simulink model "HW2_adarbha_sim"  (Simulink 7.7)
settings: Solver=ode45  StartTime=0.0  StopTime=time_end  RelTol=1e-3
PreLoadFcn:
  | HW2_adarbha
InitFcn:
  | HW2_adarbha
undefined symbols (not defined in the file): Area, Cd, density, mass, slope_deg, time_s, time_s_slope, vel_mph, weight_N
libraries: simulink x1
settings Model: Creator=Arjun  LastModifiedBy=Arjun

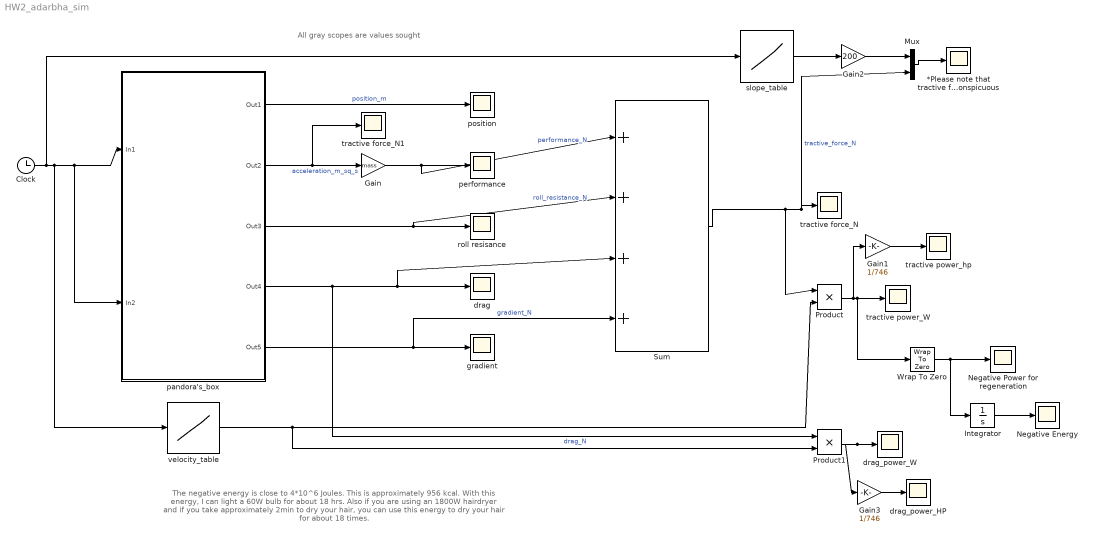
== system HW2_adarbha_sim ==
  note: The negative energy is close to 4*10^6 Joules. This is approximately 956 kcal. With this energy, I can light a 60W bulb for about 18 hrs.
      | Also if you are using an 1800W hairdryer and if you take approximately 2min to dry your hair, you can use this energy to dry your hair for about 18 times.
  note: All gray scopes are values sought
  *Please note that tractive force and slope are on the same axis but slope is multiplied by a factor of 200 so that the variation is conspicuous : Scope
      settings: SaveName=ScopeData13
  Clock : Clock
      settings: Decimation=10
  Gain : Gain  Gain=mass
  Gain1 : Gain  Gain=1/746
  Gain2 : Gain  Gain=200
  Gain3 : Gain  Gain=1/746
  Integrator : Integrator
  Mux : Mux  Inputs=2
  Negative Energy : Scope
      settings: SaveName=power_regen1  DataFormat=Array
  Negative Power for regeneration : Scope
      settings: SaveName=power_regen  DataFormat=Array
  Product : Product  RndMeth=Zero
  Product1 : Product  RndMeth=Zero
  Sum : Sum  Inputs=|++++
  Wrap To Zero : simulink/Discontinuities/Wrap To Zero  SystemSampleTime=-1  Threshold=0
  drag : Scope
      settings: SaveName=ScopeData4
  drag_power_HP : Scope
      settings: SaveName=ScopeData10
  drag_power_W : Scope
      settings: SaveName=ScopeData9
  gradient : Scope
      settings: SaveName=ScopeData5
  pandora's_box : Subsystem
  performance : Scope
      settings: SaveName=ScopeData6
  position : Scope
      settings: SaveName=ScopeData2
  roll resisance : Scope
      settings: SaveName=ScopeData3
  slope_table : Lookup_n-D  NumberOfTableDimensions=1  BreakpointsForDimension1=time_s_slope  Table=slope_deg  RndMeth=Simplest  InputSameDT=on
  tractive force_N : Scope
      settings: SaveName=ScopeData7
  tractive force_N1 : Scope
      settings: SaveName=ScopeData11
  tractive power_W : Scope
      settings: SaveName=ScopeData8
  tractive power_hp : Scope
      settings: SaveName=tractive_power  DataFormat=Array
  velocity_table : Lookup_n-D  NumberOfTableDimensions=1  BreakpointsForDimension1=time_s  Table=vel_mph  RndMeth=Simplest  InputSameDT=on
  wires:
  Clock/1 -> pandora's_box/2(In2), pandora's_box/1(In1), velocity_table/1, slope_table/1
  pandora's_box/2(Out2) -> Gain/1, tractive force_N1/1  "acceleration_m_sq_s"
  pandora's_box/1(Out1) -> position/1  "position_m"
  pandora's_box/4(Out4) -> drag/1, Sum/3, Product1/1  "drag_N"
  pandora's_box/5(Out5) -> gradient/1, Sum/4  "gradient_N"
  pandora's_box/3(Out3) -> roll resisance/1, Sum/2  "roll_resistance_N"
  Gain/1 -> performance/1, Sum/1  "performance_N"
  Sum/1 -> Product/1, tractive force_N/1, Mux/2  "tractive_force_N"
  velocity_table/1 -> Product/2, Product1/2
  Product/1 -> Gain1/1, tractive power_W/1, Wrap To Zero/1
  Product1/1 -> drag_power_W/1, Gain3/1
  Gain1/1 -> tractive power_hp/1
  Wrap To Zero/1 -> Negative Power for regeneration/1, Integrator/1
  Mux/1 -> *Please note that tractive force and slope are on the same axis but slope is multiplied by a factor of 200 so that the variation is conspicuous/1
  slope_table/1 -> Gain2/1
  Gain2/1 -> Mux/1
  Integrator/1 -> Negative Energy/1
  Gain3/1 -> drag_power_HP/1

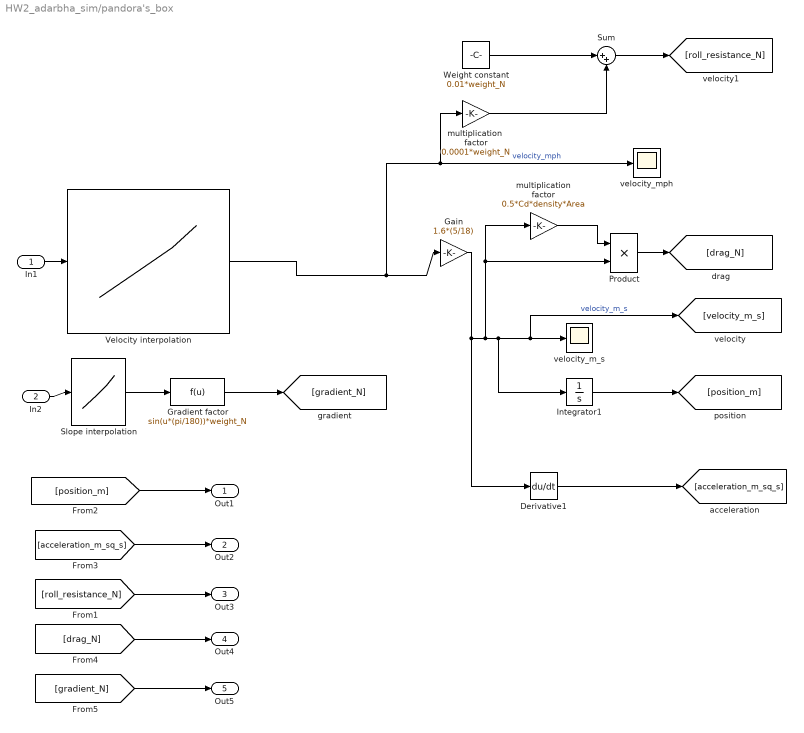
== system HW2_adarbha_sim/pandora's_box ==
  In1 : Inport
  In2 : Inport  Port=2
  Derivative1 : Derivative
  Gain : Gain  Gain=1.6*(5/18)
  Gradient factor : Fcn  Expr=sin(u*(pi/180))*weight_N
  Integrator1 : Integrator
  Product : Product  RndMeth=Zero
  Slope interpolation : Lookup_n-D  NumberOfTableDimensions=1  BreakpointsForDimension1=time_s_slope  Table=slope_deg  RndMeth=Simplest  InputSameDT=on
  Sum : Sum  Inputs=|++
  Velocity interpolation : Lookup_n-D  NumberOfTableDimensions=1  BreakpointsForDimension1=time_s  Table=vel_mph  RndMeth=Simplest  InputSameDT=on
  Weight constant : Constant  Value=0.01*weight_N
  multiplication  factor : Gain  Gain=0.0001*weight_N
  multiplication factor : Gain  Gain=0.5*Cd*density*Area
  velocity_m_s : Scope
  velocity_mph : Scope
  Out1 : Outport
  Out2 : Outport  Port=2
  Out3 : Outport  Port=3
  Out4 : Outport  Port=4
  Out5 : Outport  Port=5
  wires:
  Velocity interpolation/1 -> Gain/1, multiplication  factor/1, velocity_mph/1  "velocity_mph"
  Gain/1 -> velocity_m_s/1, [velocity_m_s], Integrator1/1, multiplication factor/1, Product/2, Derivative1/1  "velocity_m_s"
  Integrator1/1 -> [position_m]
  Derivative1/1 -> [acceleration_m_sq_s]
  [position_m] -> Out1/1
  [acceleration_m_sq_s] -> Out2/1
  Weight constant/1 -> Sum/1
  multiplication  factor/1 -> Sum/2
  Sum/1 -> [roll_resistance_N]
  [roll_resistance_N] -> Out3/1
  multiplication factor/1 -> Product/1
  Product/1 -> [drag_N]
  [drag_N] -> Out4/1
  Slope interpolation/1 -> Gradient factor/1
  Gradient factor/1 -> [gradient_N]
  [gradient_N] -> Out5/1
  In1/1 -> Velocity interpolation/1
  In2/1 -> Slope interpolation/1
